simulink model "gulocse"  (R2021a)
settings: Solver=VariableStepAuto  StartTime=0.0  StopTime=10  RelTol=1e-3
settings Model: Creator=PUGAZH  LastModifiedBy=PUGAZH

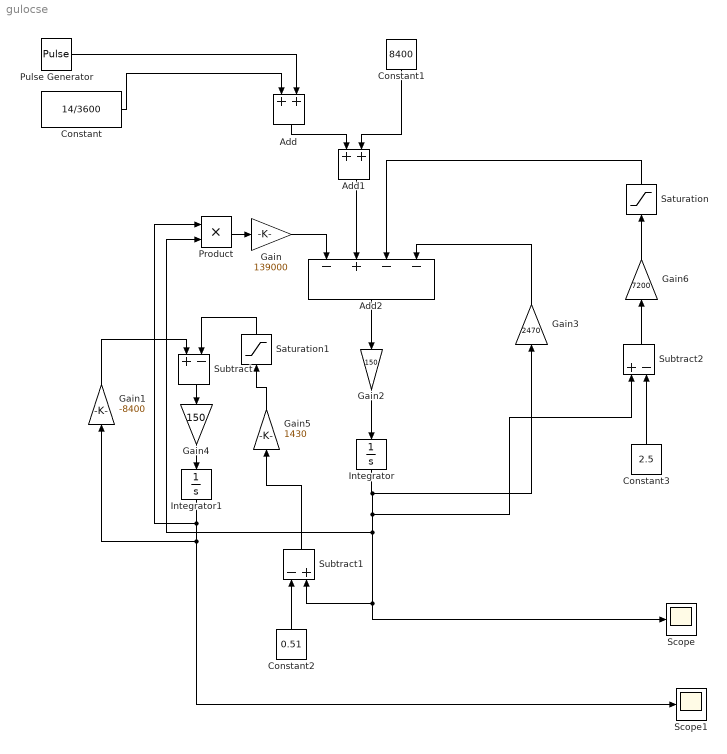
== system gulocse ==
  Add : Sum
  Add1 : Sum
  Add2 : Sum  Inputs=-+--
  Constant : Constant  Value=14/3600
  Constant1 : Constant  Value=8400
  Constant2 : Constant  Value=0.51
  Constant3 : Constant  Value=2.5
  Gain : Gain  Gain=139000
  Gain1 : Gain  Gain=-8400  ParamMax=0
  Gain2 : Gain  Gain=150
  Gain3 : Gain  Gain=2470
  Gain4 : Gain  Gain=150
  Gain5 : Gain  Gain=1430
  Gain6 : Gain  Gain=7200
  Integrator : Integrator
  Integrator1 : Integrator
  Product : Product
  Pulse Generator : DiscretePulseGenerator  PulseType=Time based  Period=10  PulseWidth=5
  Saturation : Saturate
  Saturation1 : Saturate
  Scope : Scope
  Scope1 : Scope
  Subtract : Sum  Inputs=+-
  Subtract1 : Sum  Inputs=-+
  Subtract2 : Sum  Inputs=+-
  wires:
  Constant/1 -> Add/1
  Pulse Generator/1 -> Add/2
  Add/1 -> Add1/1
  Constant1/1 -> Add1/2
  Product/1 -> Gain/1
  Gain1/1 -> Subtract/1
  Gain/1 -> Add2/1
  Add1/1 -> Add2/2
  Add2/1 -> Gain2/1
  Gain3/1 -> Add2/4
  Gain2/1 -> Integrator/1
  Integrator/1 -> Subtract2/1, Scope/1, Subtract1/2, Product/2, Gain3/1
  Subtract/1 -> Gain4/1
  Gain4/1 -> Integrator1/1
  Integrator1/1 -> Scope1/1, Gain1/1, Product/1
  Constant2/1 -> Subtract1/1
  Subtract1/1 -> Gain5/1
  Constant3/1 -> Subtract2/2
  Subtract2/1 -> Gain6/1
  Gain6/1 -> Saturation/1
  Saturation/1 -> Add2/3
  Gain5/1 -> Saturation1/1
  Saturation1/1 -> Subtract/2
